simulink model "highpass_filt"  (R2020a)
settings: Solver=VariableStepAuto  StartTime=0.0  StopTime=10.0  RelTol=1e-3
settings Model: Creator=Shubham  LastModifiedBy=Shubham

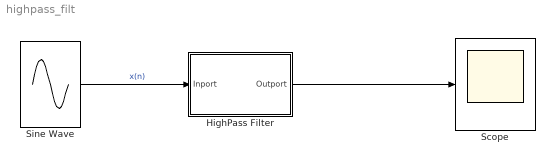
== system highpass_filt ==
  HighPass Filter : Subsystem
  Scope : Scope
  Sine Wave : Sin  SampleTime=0
  wires:
  Sine Wave/1 -> HighPass Filter/1(Inport)  "x(n)"
  HighPass Filter/1(Outport) -> Scope/1

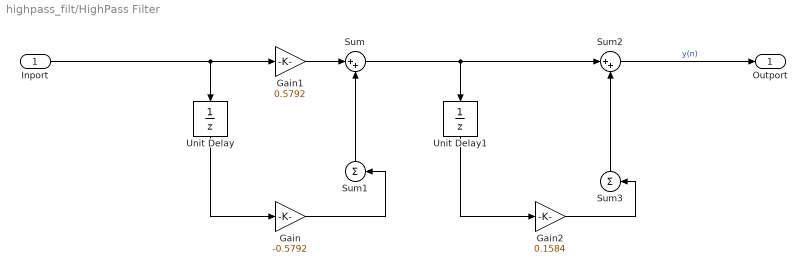
== system highpass_filt/HighPass Filter ==
  Inport : Inport
  Gain : Gain  Gain=-0.5792
  Gain1 : Gain  Gain=0.5792
  Gain2 : Gain  Gain=0.1584
  Sum : Sum  Inputs=|++
  Sum1 : Sum  Inputs=|+
  Sum2 : Sum  Inputs=|++
  Sum3 : Sum  Inputs=|+
  Unit Delay : UnitDelay  SampleTime=-1  HasFrameUpgradeWarning=on
  Unit Delay1 : UnitDelay  SampleTime=-1  HasFrameUpgradeWarning=on
  Outport : Outport
  wires:
  Inport/1 -> Unit Delay/1, Gain1/1
  Sum/1 -> Unit Delay1/1, Sum2/1
  Gain2/1 -> Sum3/1
  Sum3/1 -> Sum2/2
  Unit Delay1/1 -> Gain2/1
  Sum2/1 -> Outport/1  "y(n)"
  Sum1/1 -> Sum/2
  Unit Delay/1 -> Gain/1
  Gain1/1 -> Sum/1
  Gain/1 -> Sum1/1
